simulink model "TransitionAttributes"  (Simulink 7.4)
settings: Solver=ode45  StartTime=0.0  StopTime=10.0  RelTol=1e-3
settings Model: Creator=dread  LastModifiedBy=dread

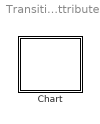
== system TransitionAttributes ==
  Chart : Stateflow chart

== stateflow chart Chart ==
  state A
  state B
  (default) -> A
  A -> B : event [true && A]
      |  {doCondition()}
      | /doTransition()
  events: event local EITHER_EDGE_EVENT
  function doCondition:
    | function doCondition
  function doTransition:
    | function doTransition
